simulink model "function_call_subsystem"  (R2021a)
settings: Solver=FixedStepAuto  StartTime=0.0  StopTime=10.0  FixedStep=1e-3  RelTol=1e-3
libraries: simulink x7
settings Model: Creator=yasso  LastModifiedBy=yasso

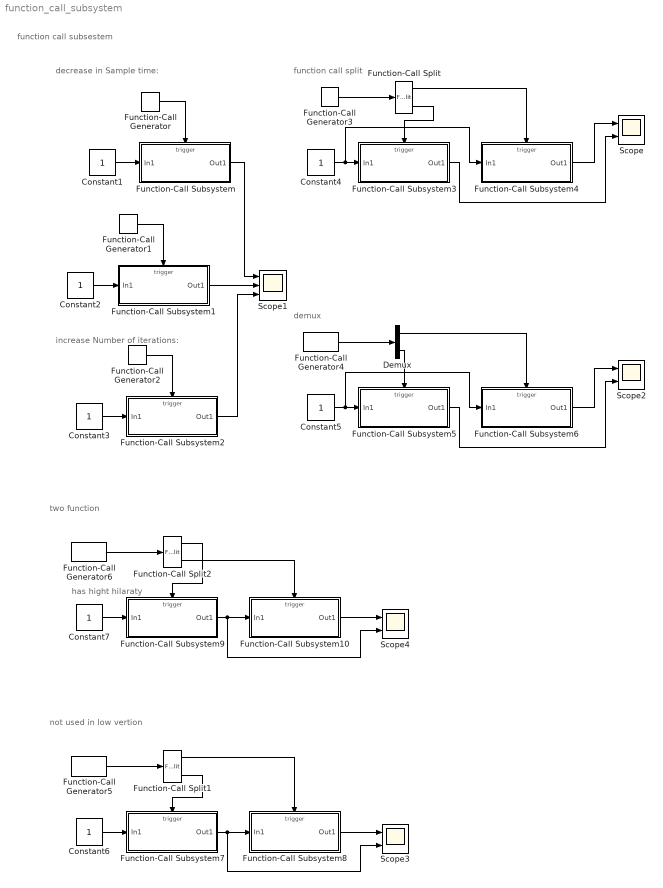
== system function_call_subsystem ==
  note: has hight hilaraty
  note: not used in low vertion
  note: function call split
  note: function call subsestem
  note: decrease in Sample time:
  note: increase Number of iterations:
  note: demux
  note: two function
  Constant{1..7} (7 alike) : Constant
  Demux : Demux  Outputs=2
  Function-Call Generator : simulink/Ports & Subsystems/Function-Call Generator  sample_time=0.1  numberOfIterations=1  DisallowWideOutput=off
  Function-Call Generator1 : simulink/Ports & Subsystems/Function-Call Generator  sample_time=1  numberOfIterations=1  DisallowWideOutput=off
  Function-Call Generator{2..6} (5 alike) : simulink/Ports & Subsystems/Function-Call Generator  sample_time=1  numberOfIterations=3  DisallowWideOutput=off
  Function-Call Split : FunctionCallSplit  IconShape=distinctive  NumOutputPorts=2  OutputPortLayout=default
  Function-Call Split1 : FunctionCallSplit  IconShape=distinctive  NumOutputPorts=2  OutputPortLayout=default
  Function-Call Split2 : FunctionCallSplit  IconShape=distinctive  NumOutputPorts=2  OutputPortLayout=default
  Function-Call Subsystem : Subsystem  TreatAsAtomicUnit=on
  Function-Call Subsystem1 : Subsystem  TreatAsAtomicUnit=on
  Function-Call Subsystem10 : Subsystem  TreatAsAtomicUnit=on
  Function-Call Subsystem2 : Subsystem  TreatAsAtomicUnit=on
  Function-Call Subsystem3 : Subsystem  TreatAsAtomicUnit=on
  Function-Call Subsystem4 : Subsystem  TreatAsAtomicUnit=on
  Function-Call Subsystem5 : Subsystem  TreatAsAtomicUnit=on
  Function-Call Subsystem6 : Subsystem  TreatAsAtomicUnit=on
  Function-Call Subsystem7 : Subsystem  TreatAsAtomicUnit=on
  Function-Call Subsystem8 : Subsystem  TreatAsAtomicUnit=on
  Function-Call Subsystem9 : Subsystem  TreatAsAtomicUnit=on
  Scope{,2..4} (4 alike) : Scope  NumInputPorts=2
  Scope1 : Scope  NumInputPorts=3
  wires:
  Constant1/1 -> Function-Call Subsystem/1(In1)
  Function-Call Generator/1 -> Function-Call Subsystem/Trigger
  Function-Call Subsystem1/1(Out1) -> Scope1/2
  Constant2/1 -> Function-Call Subsystem1/1(In1)
  Function-Call Generator1/1 -> Function-Call Subsystem1/Trigger
  Function-Call Subsystem/1(Out1) -> Scope1/1
  Function-Call Generator2/1 -> Function-Call Subsystem2/Trigger
  Constant3/1 -> Function-Call Subsystem2/1(In1)
  Function-Call Subsystem2/1(Out1) -> Scope1/3
  Constant4/1 -> Function-Call Subsystem4/1(In1), Function-Call Subsystem3/1(In1)
  Function-Call Subsystem4/1(Out1) -> Scope/1
  Function-Call Subsystem3/1(Out1) -> Scope/2
  Function-Call Generator3/1 -> Function-Call Split/1
  Function-Call Split/2 -> Function-Call Subsystem3/Trigger
  Function-Call Split/1 -> Function-Call Subsystem4/Trigger
  Demux/1 -> Function-Call Subsystem6/Trigger
  Function-Call Generator4/1 -> Demux/1
  Demux/2 -> Function-Call Subsystem5/Trigger
  Function-Call Subsystem6/1(Out1) -> Scope2/1
  Function-Call Subsystem5/1(Out1) -> Scope2/2
  Constant5/1 -> Function-Call Subsystem6/1(In1), Function-Call Subsystem5/1(In1)
  Constant6/1 -> Function-Call Subsystem7/1(In1)
  Function-Call Subsystem8/1(Out1) -> Scope3/1
  Function-Call Generator5/1 -> Function-Call Split1/1
  Function-Call Split1/1 -> Function-Call Subsystem8/Trigger
  Function-Call Subsystem7/1(Out1) -> Scope3/2, Function-Call Subsystem8/1(In1)
  Function-Call Split1/2 -> Function-Call Subsystem7/Trigger
  Function-Call Subsystem10/1(Out1) -> Scope4/1
  Function-Call Subsystem9/1(Out1) -> Scope4/2, Function-Call Subsystem10/1(In1)
  Function-Call Split2/1 -> Function-Call Subsystem9/Trigger
  Function-Call Split2/2 -> Function-Call Subsystem10/Trigger
  Constant7/1 -> Function-Call Subsystem9/1(In1)
  Function-Call Generator6/1 -> Function-Call Split2/1

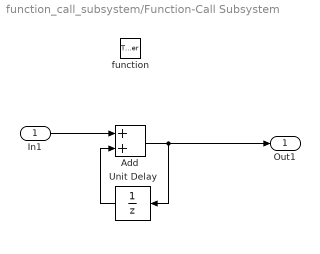
== system function_call_subsystem/Function-Call Subsystem ==
  In1 : Inport
  function : TriggerPort  TriggerType=function-call  VariantControl=(inherit)
  Add : Sum
  Unit Delay : UnitDelay  SampleTime=-1  HasFrameUpgradeWarning=on
  Out1 : Outport
  wires:
  In1/1 -> Add/1
  Add/1 -> Unit Delay/1, Out1/1
  Unit Delay/1 -> Add/2

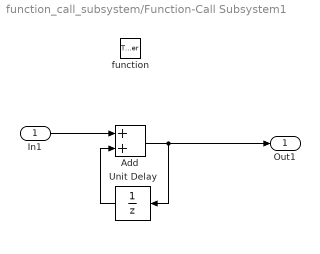
== system function_call_subsystem/Function-Call Subsystem1 ==
  In1 : Inport
  function : TriggerPort  TriggerType=function-call  VariantControl=(inherit)
  Add : Sum
  Unit Delay : UnitDelay  SampleTime=-1  HasFrameUpgradeWarning=on
  Out1 : Outport
  wires:
  In1/1 -> Add/1
  Add/1 -> Unit Delay/1, Out1/1
  Unit Delay/1 -> Add/2

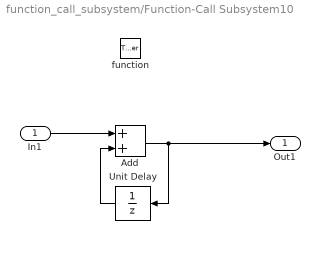
== system function_call_subsystem/Function-Call Subsystem10 ==
  In1 : Inport
  function : TriggerPort  TriggerType=function-call  VariantControl=(inherit)
  Add : Sum
  Unit Delay : UnitDelay  SampleTime=-1  HasFrameUpgradeWarning=on
  Out1 : Outport
  wires:
  In1/1 -> Add/1
  Add/1 -> Unit Delay/1, Out1/1
  Unit Delay/1 -> Add/2

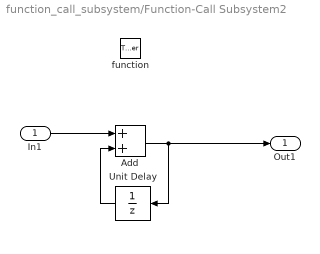
== system function_call_subsystem/Function-Call Subsystem2 ==
  In1 : Inport
  function : TriggerPort  TriggerType=function-call  VariantControl=(inherit)
  Add : Sum
  Unit Delay : UnitDelay  SampleTime=-1  HasFrameUpgradeWarning=on
  Out1 : Outport
  wires:
  Unit Delay/1 -> Add/2
  Add/1 -> Out1/1, Unit Delay/1
  In1/1 -> Add/1

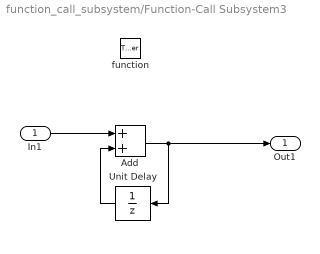
== system function_call_subsystem/Function-Call Subsystem3 ==
  In1 : Inport
  function : TriggerPort  TriggerType=function-call  VariantControl=(inherit)
  Add : Sum
  Unit Delay : UnitDelay  SampleTime=-1  HasFrameUpgradeWarning=on
  Out1 : Outport
  wires:
  Unit Delay/1 -> Add/2
  Add/1 -> Out1/1, Unit Delay/1
  In1/1 -> Add/1

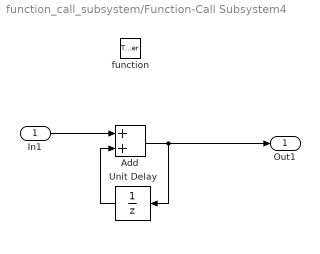
== system function_call_subsystem/Function-Call Subsystem4 ==
  In1 : Inport
  function : TriggerPort  TriggerType=function-call  VariantControl=(inherit)
  Add : Sum
  Unit Delay : UnitDelay  SampleTime=-1  HasFrameUpgradeWarning=on
  Out1 : Outport
  wires:
  In1/1 -> Add/1
  Add/1 -> Unit Delay/1, Out1/1
  Unit Delay/1 -> Add/2

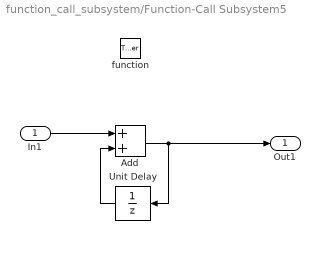
== system function_call_subsystem/Function-Call Subsystem5 ==
  In1 : Inport
  function : TriggerPort  TriggerType=function-call  VariantControl=(inherit)
  Add : Sum
  Unit Delay : UnitDelay  SampleTime=-1  HasFrameUpgradeWarning=on
  Out1 : Outport
  wires:
  Unit Delay/1 -> Add/2
  Add/1 -> Out1/1, Unit Delay/1
  In1/1 -> Add/1

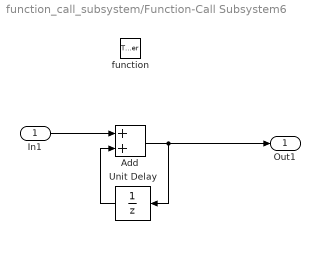
== system function_call_subsystem/Function-Call Subsystem6 ==
  In1 : Inport
  function : TriggerPort  TriggerType=function-call  VariantControl=(inherit)
  Add : Sum
  Unit Delay : UnitDelay  SampleTime=-1  HasFrameUpgradeWarning=on
  Out1 : Outport
  wires:
  In1/1 -> Add/1
  Add/1 -> Unit Delay/1, Out1/1
  Unit Delay/1 -> Add/2

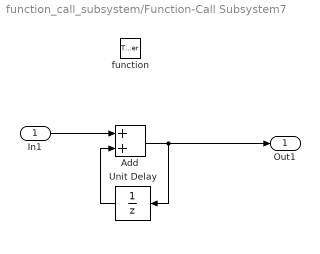
== system function_call_subsystem/Function-Call Subsystem7 ==
  In1 : Inport
  function : TriggerPort  TriggerType=function-call  VariantControl=(inherit)
  Add : Sum
  Unit Delay : UnitDelay  SampleTime=-1  HasFrameUpgradeWarning=on
  Out1 : Outport
  wires:
  Unit Delay/1 -> Add/2
  Add/1 -> Out1/1, Unit Delay/1
  In1/1 -> Add/1

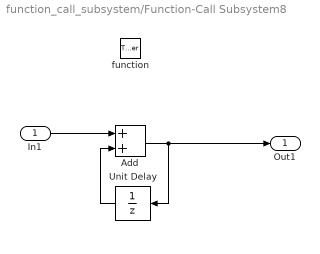
== system function_call_subsystem/Function-Call Subsystem8 ==
  In1 : Inport
  function : TriggerPort  TriggerType=function-call  VariantControl=(inherit)
  Add : Sum
  Unit Delay : UnitDelay  SampleTime=-1  HasFrameUpgradeWarning=on
  Out1 : Outport
  wires:
  In1/1 -> Add/1
  Add/1 -> Unit Delay/1, Out1/1
  Unit Delay/1 -> Add/2

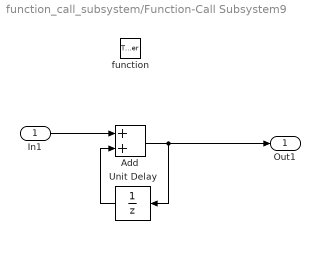
== system function_call_subsystem/Function-Call Subsystem9 ==
  In1 : Inport
  function : TriggerPort  TriggerType=function-call  VariantControl=(inherit)
  Add : Sum
  Unit Delay : UnitDelay  SampleTime=-1  HasFrameUpgradeWarning=on
  Out1 : Outport
  wires:
  Unit Delay/1 -> Add/2
  Add/1 -> Out1/1, Unit Delay/1
  In1/1 -> Add/1
